simulink model "SF003A_Dampg"  (R2013b)
settings: Solver=FixedStepDiscrete  SolverMode=SingleTasking  StartTime=0.0  StopTime=1  FixedStep=.002  RelTol=1e-3
values from neighbouring files (symbols this model uses):
  ARCHGLBPRM_2MILLISEC_SEC_F32 = DataDict.Constant    [SF003A_Dampg_DataDict.m]
  DampgHydBasCoeff1 = DataDict.Calibration    [SF003A_Dampg_DataDict.m]
  DampgHydBasCoeff2 = DataDict.Calibration    [SF003A_Dampg_DataDict.m]
  DampgHydBasCoeff3 = DataDict.Calibration    [SF003A_Dampg_DataDict.m]
  DampgHydBasCoeff4 = DataDict.Calibration    [SF003A_Dampg_DataDict.m]
  DampgHydOutpLim = DataDict.Calibration    [SF003A_Dampg_DataDict.m]
  DampgQuad13Mplr = DataDict.Calibration    [SF003A_Dampg_DataDict.m]
  DampgQuad24Mplr = DataDict.Calibration    [SF003A_Dampg_DataDict.m]
  DampgQuadHwTqBacklsh = DataDict.Calibration    [SF003A_Dampg_DataDict.m]
  DampgQuadMotVelBacklsh = DataDict.Calibration    [SF003A_Dampg_DataDict.m]
  FLTINJ_DAMPG_DAMPGCMDBAS = DataDict.Constant    [SF003A_Dampg_DataDict.m]
libraries: FloatToFixd x9, Fil x8, FixdToFloat x8, LnrIntrpn x7, NxtrAbslt x5, NxtrSign x3, NxtrLim x3, simulink x1, NxtrMax x1, BilnrIntrpnMplX x1
(part 1 of 2)
settings Model: Creator=TZ5743  LastModifiedBy=bzhf94
settings SolverCC: AutoInsertRateTranBlk=on  InsertRTBMode=Always
settings DataIOCC: LimitDataPoints=off  SaveFormat=Structure  ReturnWorkspaceOutputs=on
settings OptimizationCC: BlockReduction=off  InlineParams=on  ZeroExternalMemoryAtStartup=off  ZeroInternalMemoryAtStartup=off  OptimizeModelRefInitCode=on  LifeSpan=1
settings DebuggingCC: SignalInfNanChecking=error  SignalRangeChecking=warning  UnderspecifiedInitializationDetection=Simplified  SolverPrmCheckMsg=error  InheritedTsInSrcMsg=error  DiscreteInheritContinuousMsg=error  SingleTaskRateTransMsg=error  TasksWithSamePriorityMsg=error  SigSpecEnsureSampleTimeMsg=error  CheckMatrixSingularityMsg=error  ParameterUnderflowMsg=error  ParameterPrecisionLossMsg=error  ParameterTunabilityLossMsg=error  FixptConstUnderflowMsg=warning  FixptConstOverflowMsg=warning  VectorMatrixConversionMsg=error  SignalLabelMismatchMsg=error  UnconnectedInputMsg=error  UnconnectedOutputMsg=error  UnconnectedLineMsg=error  SFcnCompatibilityMsg=error  UniqueDataStoreMsg=warning  BusObjectLabelMismatch=error  RootOutportRequireBusObject=error  AssertControl=DisableAll  ModelReferenceIOMsg=error  ModelReferenceVersionMismatchMessage=warning  ModelReferenceIOMismatchMessage=error  ModelReferenceCSMismatchMessage=warning  ModelReferenceDataLoggingMessage=error  StateNameClashWarn=warning  StrictBusMsg=ErrorOnBusTreatedAsVector  NonBusSignalsTreatedAsBus=error  SFUnexpectedBacktrackingDiag=error  SFInvalidInputDataAccessInChartInitDiag=error  SFNoUnconditionalDefaultTransitionDiag=error  SFTransitionOutsideNaturalParentDiag=error  SFUnconditionalTransitionShadowingDiag=error  SFUndirectedBroadcastEventsDiag=error
settings ModelReferenceCC: ModelReferenceNumInstancesAllowed=Single
settings RTWCC: SystemTargetFile=autosar.tlc  GenCodeOnly=on  TemplateMakefile=ert_default_tmf  Description=AUTOSAR  GenerateReport=on  ProcessScript=autosar_make_rtw_hook  LaunchReport=on
settings CodeAppCC: GenerateComments=off  IgnoreCustomStorageClasses=off  CustomSymbolStrType=$N$R$M  CustomSymbolStrBlkIO=$N$M  SimulinkBlockComments=off
settings STFCustomTargetCC: ParMdlRefBuildCompliant=on  CompOptLevelCompliant=on  IncludeMdlTerminateFcn=off  CombineOutputUpdateFcns=on  SuppressErrorStatus=on  ERTFirstTimeCompliant=on  ERTCustomFileBanners=on  SupportNonFinite=off  SupportComplex=off  SupportContinuousTime=off  SupportNonInlinedSFcns=off  MATLABClassNameForMDSCustomization=Simulink.SoftwareTarget.ERTCustomization  AutosarCompliant=on  GRTInterface=off  SystemTargetFile=autosar.tlc
settings ERTTargetCC: CodeReplacementLibrary=ANSI_C  ConcurrentExecutionCompliant=off  IncludeMdlTerminateFcn=off  SuppressErrorStatus=on  SupportNonFinite=off  SupportComplex=off  ModelStepFunctionPrototypeControlCompliant=off  CPPClassGenCompliant=off  AutosarCompliant=on  InlinedParameterPlacement=NonHierarchical  ERTCustomFileTemplate=example_file_process.tlc  EnableUserReplacementTypes=on

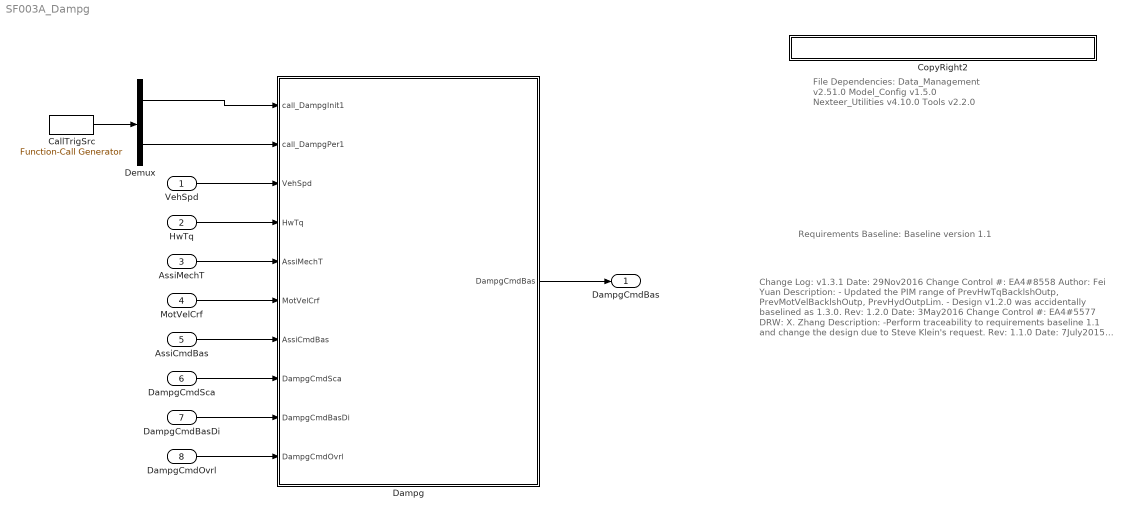
== system SF003A_Dampg ==
  note: File Dependencies:
      |
      | Data_Management v2.51.0
      | Model_Config v1.5.0
      | Nexteer_Utilities v4.10.0
      | Tools v2.2.0
  note: Requirements Baseline: Baseline version 1.1
  note: Change Log:
      |
      | v1.3.1
      | Date: 29Nov2016
      | Change Control #: EA4#8558
      | Author: Fei Yuan
      | Description:
      | - Updated the PIM range of PrevHwTqBacklshOutp,
      |   PrevMotVelBacklshOutp, PrevHydOutpLim.
      | - Design v1.2.0 was accidentally baselined as 1.3.0.
      |
      |
      | Rev: 1.2.0
      | Date: 3May2016
      | Change Control #: EA4#5577
      | DRW: X. Zhang
      | Description:
      | -Perform traceability to requirements baseline 1.1
      | and change the design due to Steve Klein's request.
      |
      | Rev: 1.1.0
      | Date: 7July2015
      | Change Control #: EA4#762
      | DRW: Sudeep Shankar
      | Description:
      | - Design update from EA3 to EA4 with data dictionary
      | changes.
      |
      |
      | v1.0.0
      | Date: 24-Jun-2015
      | Change Control #: EA4#762
      | DRW:  Sudeep Shankar
      | Description:
      | - Initial Release based off of EA3 Version 009
  VehSpd : Inport  RequirementInfo={'linktype_rmi_doors' '0000a525 (/E-STEER Core/SubSystem Specifications/Application Functions/SF003A Damping)' '#SF003A_33' 'true' 'REQ: SF003A_33' '' } %GIDa_568c51fe_83b0_458b_bd6e_4be12eab579e
  HwTq : Inport  RequirementInfo={'linktype_rmi_doors' '0000a525 (/E-STEER Core/SubSystem Specifications/Application Functions/SF003A Damping)' '#SF003A_34' 'true' 'REQ: SF003A_34' '' } %GIDa_93ae967a_0df1_4d53_9d75_79742e7754a9  Port=2
  AssiMechT : Inport  RequirementInfo={'linktype_rmi_doors' '0000a525 (/E-STEER Core/SubSystem Specifications/Application Functions/SF003A Damping)' '#SF003A_35' 'true' 'REQ: SF003A_35' '' } %GIDa_1636facc_5bec_431d_9ade_0f003592cb00  Port=3
  MotVelCrf : Inport  RequirementInfo={'linktype_rmi_doors' '0000a525 (/E-STEER Core/SubSystem Specifications/Application Functions/SF003A Damping)' '#SF003A_36' 'true' 'REQ: SF003A_36' '' } %GIDa_f33306b7_8b32_4dca_8a0a_81a3a24a2a49  Port=4
  AssiCmdBas : Inport  RequirementInfo={'linktype_rmi_doors' '0000a525 (/E-STEER Core/SubSystem Specifications/Application Functions/SF003A Damping)' '#SF003A_37' 'true' 'REQ: SF003A_37' '' } %GIDa_bfde9b7a_b609_47ac_97d9_497bdc083739  Port=5
  DampgCmdSca : Inport  RequirementInfo={'linktype_rmi_doors' '0000a525 (/E-STEER Core/SubSystem Specifications/Application Functions/SF003A Damping)' '#SF003A_38' 'true' 'REQ: SF003A_38' '' } %GIDa_3f9e7f26_4227_4164_8f57_da4171e42017  Port=6
  DampgCmdBasDi : Inport  RequirementInfo={'linktype_rmi_doors' '0000a525 (/E-STEER Core/SubSystem Specifications/Application Functions/SF003A Damping)' '#SF003A_9' 'true' 'REQ: SF003A_9' '' } %GIDa_728ec3ad_7cb0_4a0a_ae43_e264b5abcd56  Port=7
  DampgCmdOvrl : Inport  RequirementInfo={'linktype_rmi_doors' '0000a525 (/E-STEER Core/SubSystem Specifications/Application Functions/SF003A Damping)' '#SF003A_63' 'true' 'REQ: SF003A_63' '' } %GIDa_4827e2e0_a4cb_4f02_b938_6d875c7b4f9b  Port=8
  CallTrigSrc : simulink/Ports & Subsystems/Function-Call Generator  RequirementInfo={} %GIDa_ba0e12fc_4474_4f55_8217_81b6c7a3534f  sample_time=0.002  numberOfIterations=1
  CopyRight2 : Subsystem  Description=|  mask(Copyright Information){none=on}
      | Copyright info block.                                               
      |                                                                     
      | Place copyright information at the top of every subsystem in design.
      mask prompts: none "No parameters"
      mask help: Place copyright information at the top of every subsystem in design.
      mask Display:
      | NxtrConf = 'Nexteer Confidential';
      | 
      | sys = bdroot; %handle for the current model ("system")
      | first = get_param(sys,'Created');
      | if(isempty(first))
      |     first = datestr(now,'yyyy');
      | else
      |     first = first(end-3:end);  %year is last four digits
      | end
      | 
      | last = get_param(sys,'LastModifiedDate');
      | if isempty(last)
      |     last = datestr(now,'yyyy');
      | else
      |     last = last(end-3:end);
      | end
      | 
      | if strcmp(first,last)
      |     fprintf('%s -- Copyright %s Nexteer',NxtrConf,first)
      | else
      |     fprintf('%s -- %s%s- %s Nexteer',NxtrConf,char(169),first,last)
      | end
  Dampg : Subsystem
  Demux : Demux  Outputs=2
  DampgCmdBas : Outport  RequirementInfo={'linktype_rmi_doors' '0000a525 (/E-STEER Core/SubSystem Specifications/Application Functions/SF003A Damping)' '#SF003A_11' 'true' 'REQ: SF003A_11' '' } %GIDa_820641fa_7a17_4c33_aa73_2ea523178ec1
  wires:
  Demux/2 -> Dampg/2(call_DampgPer1)
  VehSpd/1 -> Dampg/3(VehSpd)
  HwTq/1 -> Dampg/4(HwTq)
  AssiMechT/1 -> Dampg/5(AssiMechT)
  MotVelCrf/1 -> Dampg/6(MotVelCrf)
  AssiCmdBas/1 -> Dampg/7(AssiCmdBas)
  DampgCmdSca/1 -> Dampg/8(DampgCmdSca)
  DampgCmdBasDi/1 -> Dampg/9(DampgCmdBasDi)
  DampgCmdOvrl/1 -> Dampg/10(DampgCmdOvrl)
  Dampg/1(DampgCmdBas) -> DampgCmdBas/1
  CallTrigSrc/1 -> Demux/1
  Demux/1 -> Dampg/1(call_DampgInit1)

== system SF003A_Dampg/CopyRight2 ==

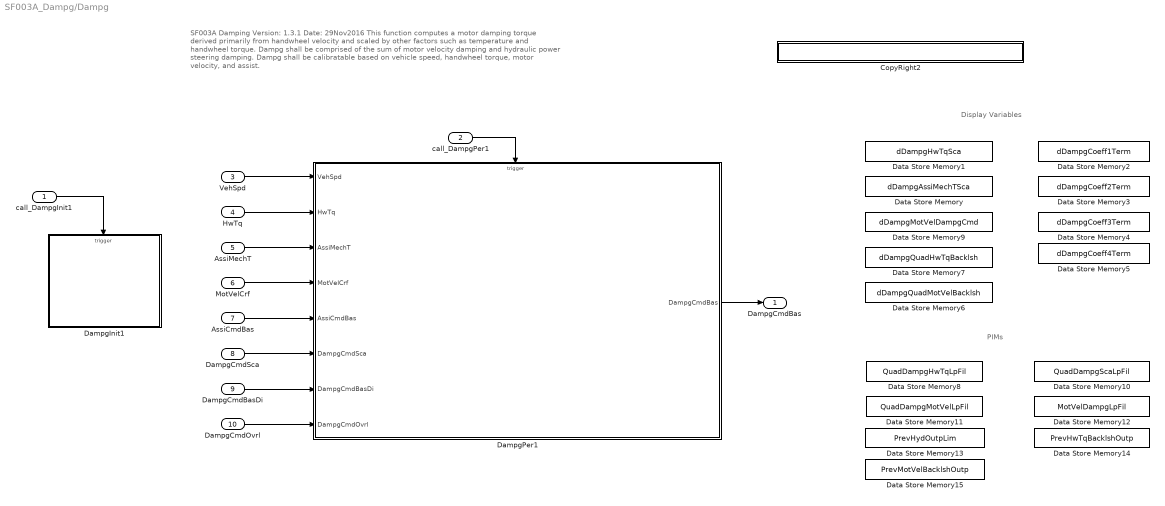
== system SF003A_Dampg/Dampg ==
  note: PIMs
  note: Display Variables
  note: SF003A Damping       Version: 1.3.1                                                      Date: 29Nov2016
      |
      | This function computes a motor damping torque derived primarily from handwheel velocity and scaled by other factors such as temperature and handwheel torque.
      | Dampg shall be comprised of the sum of motor velocity damping and hydraulic power steering damping.
      | Dampg shall be calibratable based on vehicle speed, handwheel torque, motor velocity, and assist.
  call_DampgInit1 : Inport
  call_DampgPer1 : Inport  Port=2
  VehSpd : Inport  Port=3
  HwTq : Inport  Port=4
  AssiMechT : Inport  Port=5
  MotVelCrf : Inport  Port=6
  AssiCmdBas : Inport  Port=7
  DampgCmdSca : Inport  Port=8
  DampgCmdBasDi : Inport  Port=9
  DampgCmdOvrl : Inport  Port=10
  CopyRight2 : Subsystem  Description=|  mask(Copyright Information){none=on}
      | Copyright info block.                                               
      |                                                                     
      | Place copyright information at the top of every subsystem in design.
      mask prompts: none "No parameters"
      mask help: Place copyright information at the top of every subsystem in design.
      mask Display:
      | NxtrConf = 'Nexteer Confidential';
      | 
      | sys = bdroot; %handle for the current model ("system")
      | first = get_param(sys,'Created');
      | if(isempty(first))
      |     first = datestr(now,'yyyy');
      | else
      |     first = first(end-3:end);  %year is last four digits
      | end
      | 
      | last = get_param(sys,'LastModifiedDate');
      | if isempty(last)
      |     last = datestr(now,'yyyy');
      | else
      |     last = last(end-3:end);
      | end
      | 
      | if strcmp(first,last)
      |     fprintf('%s -- Copyright %s Nexteer',NxtrConf,first)
      | else
      |     fprintf('%s -- %s%s- %s Nexteer',NxtrConf,char(169),first,last)
      | end
  DampgInit1 : Subsystem
  DampgPer1 : Subsystem
  Data Store Memory : DataStoreMemory  DataStoreName=dDampgAssiMechTSca  ReadBeforeWriteMsg=warning  WriteAfterWriteMsg=warning  WriteAfterReadMsg=warning  StateMustResolveToSignalObject=on
  Data Store Memory1 : DataStoreMemory  DataStoreName=dDampgHwTqSca  ReadBeforeWriteMsg=warning  WriteAfterWriteMsg=warning  WriteAfterReadMsg=warning  OutDataTypeStr=single  StateMustResolveToSignalObject=on
  Data Store Memory10 : DataStoreMemory  DataStoreName=QuadDampgScaLpFil  InitialValue=struct('FilSt',single(0),'FilGain',single(0))  OutDataTypeStr=Bus: FilLpRec1  StateMustResolveToSignalObject=on
  Data Store Memory11 : DataStoreMemory  DataStoreName=QuadDampgMotVelLpFil  InitialValue=struct('FilSt',single(0),'FilGain',single(0))  OutDataTypeStr=Bus: FilLpRec1  StateMustResolveToSignalObject=on
  Data Store Memory12 : DataStoreMemory  DataStoreName=MotVelDampgLpFil  InitialValue=struct('FilSt',single(0),'FilGain',single(0))  OutDataTypeStr=Bus: FilLpRec1  StateMustResolveToSignalObject=on
  Data Store Memory13 : DataStoreMemory  DataStoreName=PrevHydOutpLim  StateMustResolveToSignalObject=on
  Data Store Memory14 : DataStoreMemory  DataStoreName=PrevHwTqBacklshOutp  StateMustResolveToSignalObject=on
  Data Store Memory15 : DataStoreMemory  DataStoreName=PrevMotVelBacklshOutp  StateMustResolveToSignalObject=on
  Data Store Memory2 : DataStoreMemory  DataStoreName=dDampgCoeff1Term  ReadBeforeWriteMsg=warning  WriteAfterWriteMsg=warning  WriteAfterReadMsg=warning  OutDataTypeStr=single  StateMustResolveToSignalObject=on
  Data Store Memory3 : DataStoreMemory  DataStoreName=dDampgCoeff2Term  ReadBeforeWriteMsg=warning  WriteAfterWriteMsg=warning  WriteAfterReadMsg=warning  OutDataTypeStr=single  StateMustResolveToSignalObject=on
  Data Store Memory4 : DataStoreMemory  DataStoreName=dDampgCoeff3Term  ReadBeforeWriteMsg=warning  WriteAfterWriteMsg=warning  WriteAfterReadMsg=warning  OutDataTypeStr=single  StateMustResolveToSignalObject=on
  Data Store Memory5 : DataStoreMemory  DataStoreName=dDampgCoeff4Term  ReadBeforeWriteMsg=warning  WriteAfterWriteMsg=warning  WriteAfterReadMsg=warning  OutDataTypeStr=single  StateMustResolveToSignalObject=on
  Data Store Memory6 : DataStoreMemory  DataStoreName=dDampgQuadMotVelBacklsh  ReadBeforeWriteMsg=warning  WriteAfterWriteMsg=warning  WriteAfterReadMsg=warning  StateMustResolveToSignalObject=on
  Data Store Memory7 : DataStoreMemory  DataStoreName=dDampgQuadHwTqBacklsh  ReadBeforeWriteMsg=warning  WriteAfterWriteMsg=warning  WriteAfterReadMsg=warning  StateMustResolveToSignalObject=on
  Data Store Memory8 : DataStoreMemory  DataStoreName=QuadDampgHwTqLpFil  InitialValue=struct('FilSt',single(0),'FilGain',single(0))  OutDataTypeStr=Bus: FilLpRec1  StateMustResolveToSignalObject=on
  Data Store Memory9 : DataStoreMemory  DataStoreName=dDampgMotVelDampgCmd  ReadBeforeWriteMsg=warning  WriteAfterWriteMsg=warning  WriteAfterReadMsg=warning  StateMustResolveToSignalObject=on
  DampgCmdBas : Outport
  wires:
  MotVelCrf/1 -> DampgPer1/4(MotVelCrf)
  DampgCmdBasDi/1 -> DampgPer1/7(DampgCmdBasDi)
  DampgPer1/1(DampgCmdBas) -> DampgCmdBas/1
  DampgCmdSca/1 -> DampgPer1/6(DampgCmdSca)
  AssiMechT/1 -> DampgPer1/3(AssiMechT)
  DampgCmdOvrl/1 -> DampgPer1/8(DampgCmdOvrl)
  HwTq/1 -> DampgPer1/2(HwTq)
  AssiCmdBas/1 -> DampgPer1/5(AssiCmdBas)
  VehSpd/1 -> DampgPer1/1(VehSpd)
  call_DampgPer1/1 -> DampgPer1/Trigger
  call_DampgInit1/1 -> DampgInit1/Trigger

== system SF003A_Dampg/Dampg/CopyRight2 ==

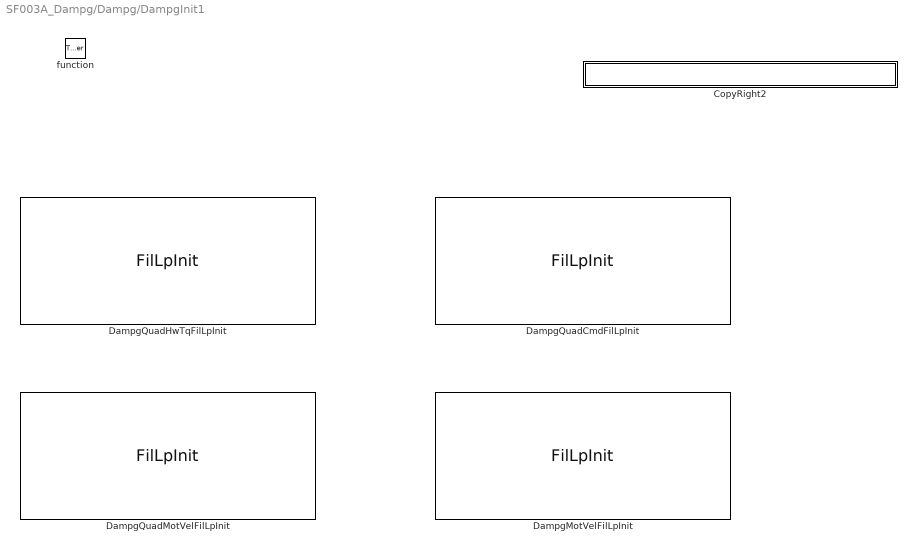
== system SF003A_Dampg/Dampg/DampgInit1 ==
  function : TriggerPort  TriggerType=function-call
  CopyRight2 : Subsystem  Description=|  mask(Copyright Information){none=on}
      | Copyright info block.                                               
      |                                                                     
      | Place copyright information at the top of every subsystem in design.
      mask prompts: none "No parameters"
      mask help: Place copyright information at the top of every subsystem in design.
      mask Display:
      | NxtrConf = 'Nexteer Confidential';
      | 
      | sys = bdroot; %handle for the current model ("system")
      | first = get_param(sys,'Created');
      | if(isempty(first))
      |     first = datestr(now,'yyyy');
      | else
      |     first = first(end-3:end);  %year is last four digits
      | end
      | 
      | last = get_param(sys,'LastModifiedDate');
      | if isempty(last)
      |     last = datestr(now,'yyyy');
      | else
      |     last = last(end-3:end);
      | end
      | 
      | if strcmp(first,last)
      |     fprintf('%s -- Copyright %s Nexteer',NxtrConf,first)
      | else
      |     fprintf('%s -- %s%s- %s Nexteer',NxtrConf,char(169),first,last)
      | end
  DampgMotVelFilLpInit : Fil/FilLpInit  Ic=0  Ts=ARCHGLBPRM_2MILLISEC_SEC_F32  Freq=DampgMotVelLpFilFrq  StVar=MotVelDampgLpFil
  DampgQuadCmdFilLpInit : Fil/FilLpInit  Ic=0  Ts=ARCHGLBPRM_2MILLISEC_SEC_F32  Freq=DampgQuadScaLpFilFrq  StVar=QuadDampgScaLpFil
  DampgQuadHwTqFilLpInit : Fil/FilLpInit  Ic=0  Ts=ARCHGLBPRM_2MILLISEC_SEC_F32  Freq=DampgQuadHwTqLpFilFrq  StVar=QuadDampgHwTqLpFil
  DampgQuadMotVelFilLpInit : Fil/FilLpInit  Ic=0  Ts=ARCHGLBPRM_2MILLISEC_SEC_F32  Freq=DampgQuadMotVelLpFilFrq  StVar=QuadDampgMotVelLpFil

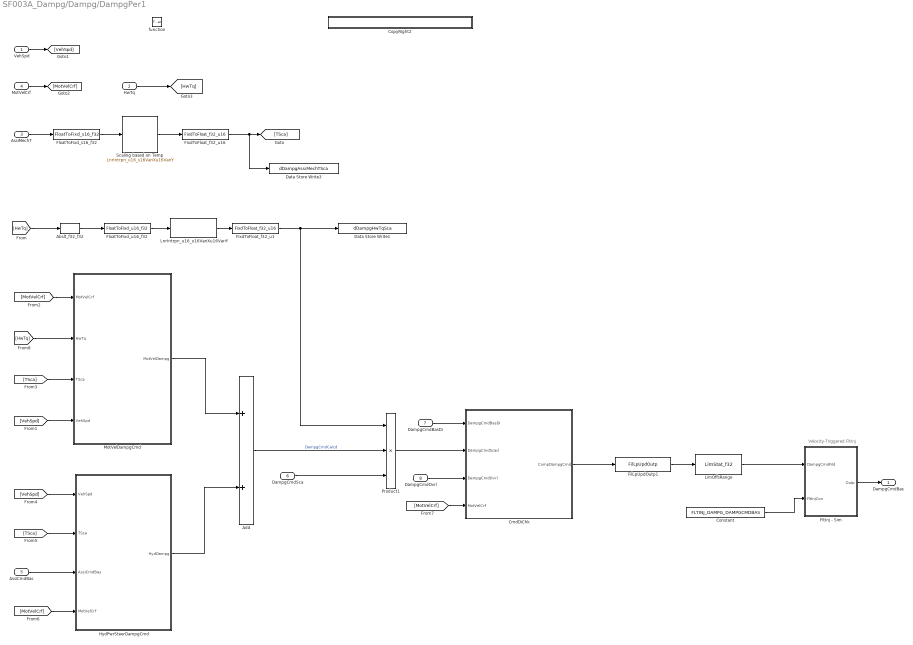
== system SF003A_Dampg/Dampg/DampgPer1 ==
  note: Velocity-Triggered FltInj
  VehSpd : Inport
  HwTq : Inport  Port=2
  AssiMechT : Inport  RequirementInfo={'linktype_rmi_doors' '0000a525 (/E-STEER Core/SubSystem Specifications/Application Functions/SF003A Damping)' '#SF003A_83' 'true' 'REQ: SF003A_83' '' } %GIDa_7550e755_adaf_43cd_af46_c12af1f44501  Port=3
  MotVelCrf : Inport  Port=4
  AssiCmdBas : Inport  Port=5
  DampgCmdSca : Inport  Port=6
  DampgCmdBasDi : Inport  Port=7
  DampgCmdOvrl : Inport  Port=8
  function : TriggerPort  TriggerType=function-call
  Abslt_f32_f32 : NxtrAbslt/Abslt_f32_f32  RequirementInfo={'linktype_rmi_doors' '0000a525 (/E-STEER Core/SubSystem Specifications/Application Functions/SF003A Damping)' '#SF003A_93' 'true' 'REQ: SF003A_93' '' } %GIDa_152aa55c_ff3e_4795_aeae_1a4fd5587628  SFunctionSpec=single y1 = Abslt_f32_f32(single u1)
      settings: AttributesFormatString=%<Name>
  Add : Sum  RequirementInfo={'linktype_rmi_doors' '0000a525 (/E-STEER Core/SubSystem Specifications/Application Functions/SF003A Damping)' '#SF003A_125' 'true' 'REQ: SF003A_125' '' } %GIDa_a51e37c2_da29_4b95_a7c8_8c19c8d9e4f2
  CmdDiChk : Subsystem
  Constant : Constant  Value=FLTINJ_DAMPG_DAMPGCMDBAS
  CopyRight2 : Subsystem  Description=|  mask(Copyright Information){none=on}
      | Copyright info block.                                               
      |                                                                     
      | Place copyright information at the top of every subsystem in design.
      mask prompts: none "No parameters"
      mask help: Place copyright information at the top of every subsystem in design.
      mask Display:
      | NxtrConf = 'Nexteer Confidential';
      | 
      | sys = bdroot; %handle for the current model ("system")
      | first = get_param(sys,'Created');
      | if(isempty(first))
      |     first = datestr(now,'yyyy');
      | else
      |     first = first(end-3:end);  %year is last four digits
      | end
      | 
      | last = get_param(sys,'LastModifiedDate');
      | if isempty(last)
      |     last = datestr(now,'yyyy');
      | else
      |     last = last(end-3:end);
      | end
      | 
      | if strcmp(first,last)
      |     fprintf('%s -- Copyright %s Nexteer',NxtrConf,first)
      | else
      |     fprintf('%s -- %s%s- %s Nexteer',NxtrConf,char(169),first,last)
      | end
  Data Store Write1 : DataStoreWrite  DataStoreName=dDampgHwTqSca
  Data Store Write3 : DataStoreWrite  DataStoreName=dDampgAssiMechTSca
  FilLpUpdOutp1 : Fil/FilLpUpdOutp  RequirementInfo={'linktype_rmi_doors' '0000a525 (/E-STEER Core/SubSystem Specifications/Application Functions/SF003A Damping)' '#SF003A_130' 'true' 'REQ: SF003A_130' '' } %GIDa_9b76992c_6716_46d2_8232_6364667a20c4  StVar=MotVelDampgLpFil
      settings: AttributesFormatString=StVar: %<StVar>
  FixdToFloat_f32_u1 : FixdToFloat/FixdToFloat_f32_u16  RequirementInfo={'linktype_rmi_doors' '0000a525 (/E-STEER Core/SubSystem Specifications/Application Functions/SF003A Damping)' '#SF003A_93' 'true' 'REQ: SF003A_93' '' } %GIDa_93b5cec2_bcdc_4944_b939_7a0cd5e9fed0  Param1=15
  FixdToFloat_f32_u16 : FixdToFloat/FixdToFloat_f32_u16  RequirementInfo={'linktype_rmi_doors' '0000a525 (/E-STEER Core/SubSystem Specifications/Application Functions/SF003A Damping)' '#SF003A_83' 'true' 'REQ: SF003A_83' '' } %GIDa_983a16aa_5c94_4ecb_93d6_d25a8d58e50a  Param1=12
  FloatToFixd_s16_f32 : FloatToFixd/FloatToFixd_s16_f32  RequirementInfo={'linktype_rmi_doors' '0000a525 (/E-STEER Core/SubSystem Specifications/Application Functions/SF003A Damping)' '#SF003A_83' 'true' 'REQ: SF003A_83' '' } %GIDa_f83f1ff1_03e3_4238_8bb3_25bc87451b9b  Param1=7
  FloatToFixd_u16_f32 : FloatToFixd/FloatToFixd_u16_f32  RequirementInfo={'linktype_rmi_doors' '0000a525 (/E-STEER Core/SubSystem Specifications/Application Functions/SF003A Damping)' '#SF003A_93' 'true' 'REQ: SF003A_93' '' } %GIDa_9d01660a_d186_40b6_83ad_ef8a565f4b3d  Param1=8
  FltInj - Sim : Subsystem  TreatAsAtomicUnit=on  VariantControl=FltInj_sim  mask(Fault_Injection){}
      mask help: Fault Injection is a simulation only block for EA4 programs.
  HydPwrSteerDampgCmd : Subsystem
  LimOffsRange : NxtrLim/LimStat_f32  RequirementInfo={'linktype_rmi_doors' '0000a525 (/E-STEER Core/SubSystem Specifications/Application Functions/SF003A Damping)' '#SF003A_131' 'true' 'REQ: SF003A_131' '' } %GIDa_822a07d5_0f05_4298_8afc_97f880dca36e  LoLim=SYSGLBPRM_MOTTQCMDLOLIM_MOTNWTMTR_F32  HiLim=SYSGLBPRM_MOTTQCMDHILIM_MOTNWTMTR_F32
      settings: AttributesFormatString=|
      | Low Limit: %<LoLim>
      | High Limit:%<HiLim>
  LnrIntrpn_u16_u16VariXu16VariY : LnrIntrpn/LnrIntrpn_u16_u16VariXu16VariY  RequirementInfo={'linktype_rmi_doors' '0000a525 (/E-STEER Core/SubSystem Specifications/Application Functions/SF003A Damping)' '#SF003A_93' 'true' 'REQ: SF003A_93' '' } %GIDa_b3e63933_aa2e_4fdf_a46c_c146a010da00  XTbl=DampgHwTqX  YTbl=DampgHwTqY
      settings: AttributesFormatString=Lnr ( u16VariX , u16VariY )
  MotVelDampgCmd : Subsystem
  Product1 : Product  RequirementInfo={'linktype_rmi_doors' '0000a525 (/E-STEER Core/SubSystem Specifications/Application Functions/SF003A Damping)' '#SF003A_126' 'true' 'REQ: SF003A_126' '' } %GIDa_ea32ba7a_0ccc_4c1b_8193_7b5dfbd1e212  Inputs=3  RndMeth=Zero
  Scaling based on Temp : LnrIntrpn/LnrIntrpn_u16_s16VariXu16VariY  RequirementInfo={'linktype_rmi_doors' '0000a525 (/E-STEER Core/SubSystem Specifications/Application Functions/SF003A Damping)' '#SF003A_83' 'true' 'REQ: SF003A_83' '' } %GIDa_d6c5a0d2_c9b9_4dbb_9c7f_b096228439d7  XTbl=DampgTScaX  YTbl=DampgTScaY
      settings: AttributesFormatString=Lnr ( s16VariX , u16VariY )
  DampgCmdBas : Outport
  wires:
  Constant/1 -> FltInj - Sim/2(FltInjCon)
  FltInj - Sim/1(Outp) -> DampgCmdBas/1
  Product1/1 -> CmdDiChk/2(DampgCmdScad)
  CmdDiChk/1(CompDampgCmd) -> FilLpUpdOutp1/1
  DampgCmdOvrl/1 -> CmdDiChk/3(DampgCmdOvrl)
  DampgCmdBasDi/1 -> CmdDiChk/1(DampgCmdBasDi)
  LimOffsRange/1 -> FltInj - Sim/1(DampgCmdFild)
  Scaling based on Temp/1 -> FixdToFloat_f32_u16/1
  AssiMechT/1 -> FloatToFixd_s16_f32/1
  FloatToFixd_s16_f32/1 -> Scaling based on Temp/1
  FixdToFloat_f32_u16/1 -> Data Store Write3/1, [TSca]
  VehSpd/1 -> [VehSpd]
  MotVelCrf/1 -> [MotVelCrf]
  [MotVelCrf] -> MotVelDampgCmd/1(MotVelCrf)
  [VehSpd] -> MotVelDampgCmd/4(VehSpd)
  [TSca] -> MotVelDampgCmd/3(TSca)
  [VehSpd] -> HydPwrSteerDampgCmd/1(VehSpd)
  [TSca] -> HydPwrSteerDampgCmd/2(TSca)
  AssiCmdBas/1 -> HydPwrSteerDampgCmd/3(AssiCmdBas)
  [MotVelCrf] -> HydPwrSteerDampgCmd/4(MotVelCrf)
  HydPwrSteerDampgCmd/1(HydDampg) -> Add/2
  MotVelDampgCmd/1(MotVelDampg) -> Add/1
  Add/1 -> Product1/2  "DampgCmdCalcd"
  DampgCmdSca/1 -> Product1/3
  [MotVelCrf] -> CmdDiChk/4(MotVelCrf)
  FilLpUpdOutp1/1 -> LimOffsRange/1
  FloatToFixd_u16_f32/1 -> LnrIntrpn_u16_u16VariXu16VariY/1
  LnrIntrpn_u16_u16VariXu16VariY/1 -> FixdToFloat_f32_u1/1
  FixdToFloat_f32_u1/1 -> Product1/1, Data Store Write1/1
  Abslt_f32_f32/1 -> FloatToFixd_u16_f32/1
  HwTq/1 -> [HwTq]
  [HwTq] -> Abslt_f32_f32/1
  [HwTq] -> MotVelDampgCmd/2(HwTq)

== system SF003A_Dampg/Dampg/DampgInit1/CopyRight2 ==

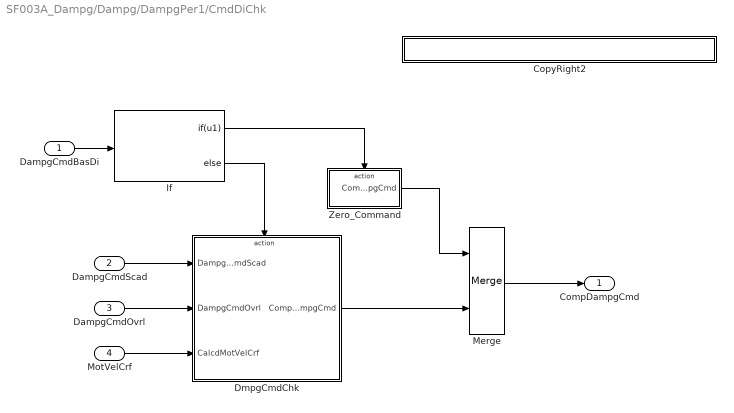
== system SF003A_Dampg/Dampg/DampgPer1/CmdDiChk ==
  DampgCmdBasDi : Inport
  DampgCmdScad : Inport  Port=2
  DampgCmdOvrl : Inport  Port=3
  MotVelCrf : Inport  Port=4
  CopyRight2 : Subsystem  Description=|  mask(Copyright Information){none=on}
      | Copyright info block.                                               
      |                                                                     
      | Place copyright information at the top of every subsystem in design.
      mask prompts: none "No parameters"
      mask help: Place copyright information at the top of every subsystem in design.
      mask Display:
      | NxtrConf = 'Nexteer Confidential';
      | 
      | sys = bdroot; %handle for the current model ("system")
      | first = get_param(sys,'Created');
      | if(isempty(first))
      |     first = datestr(now,'yyyy');
      | else
      |     first = first(end-3:end);  %year is last four digits
      | end
      | 
      | last = get_param(sys,'LastModifiedDate');
      | if isempty(last)
      |     last = datestr(now,'yyyy');
      | else
      |     last = last(end-3:end);
      | end
      | 
      | if strcmp(first,last)
      |     fprintf('%s -- Copyright %s Nexteer',NxtrConf,first)
      | else
      |     fprintf('%s -- %s%s- %s Nexteer',NxtrConf,char(169),first,last)
      | end
  DmpgCmdChk : Subsystem  RequirementInfo={} %GIDa_42609f80_721e_4222_a854_978db5b32e82  TreatAsAtomicUnit=on
  If : If  RequirementInfo={} %GIDa_e8daf89a_735d_4ce3_8883_6d943d5da402  IfExpression=u1
  Merge : Merge
  Zero_Command : Subsystem  RequirementInfo={'linktype_rmi_doors' '0000a525 (/E-STEER Core/SubSystem Specifications/Application Functions/SF003A Damping)' '#SF003A_127' 'true' 'REQ: SF003A_127' '' } %GIDa_8150363f_e871_4e58_837a_c9fd5c39bb6f  TreatAsAtomicUnit=on
  CompDampgCmd : Outport
  wires:
  If/2 -> DmpgCmdChk/Action
  If/1 -> Zero_Command/Action
  DampgCmdScad/1 -> DmpgCmdChk/1(DampgCmdScad)
  DmpgCmdChk/1(CompDampgCmd) -> Merge/2
  Zero_Command/1(CompDampgCmd) -> Merge/1
  Merge/1 -> CompDampgCmd/1
  DampgCmdBasDi/1 -> If/1
  DampgCmdOvrl/1 -> DmpgCmdChk/2(DampgCmdOvrl)
  MotVelCrf/1 -> DmpgCmdChk/3(CalcdMotVelCrf)

== system SF003A_Dampg/Dampg/DampgPer1/CopyRight2 ==

== system SF003A_Dampg/Dampg/DampgPer1/FltInj - Sim ==
  note: Inport #2 must be Constant
  note: EA4.x Fault Injection
  note: This block requires no modification by FDD author.
      |
      | This block does not actually simulate any fault injection.  It is simply a pass-thru.
      |
      | The port (#2) simply terminates its signal, but we are trying to force the FDD author
      | to properly use the Constant in FDD model.
  DampgCmdFild : Inport
  FltInjCon : Inport  Port=2
  CopyRight2 : Subsystem  Description=|  mask(Copyright Information){none=on}
      | Copyright info block.                                               
      |                                                                     
      | Place copyright information at the top of every subsystem in design.
      mask prompts: none "No parameters"
      mask help: Place copyright information at the top of every subsystem in design.
      mask Display:
      | NxtrConf = 'Nexteer Confidential';
      | 
      | sys = bdroot; %handle for the current model ("system")
      | first = get_param(sys,'Created');
      | if(isempty(first))
      |     first = datestr(now,'yyyy');
      | else
      |     first = first(end-3:end);  %year is last four digits
      | end
      | 
      | last = get_param(sys,'LastModifiedDate');
      | if isempty(last)
      |     last = datestr(now,'yyyy');
      | else
      |     last = last(end-3:end);
      | end
      | 
      | if strcmp(first,last)
      |     fprintf('%s -- Copyright %s Nexteer',NxtrConf,first)
      | else
      |     fprintf('%s -- %s%s- %s Nexteer',NxtrConf,char(169),first,last)
      | end
  Terminator : Terminator
  Outp : Outport
  wires:
  FltInjCon/1 -> Terminator/1
  DampgCmdFild/1 -> Outp/1

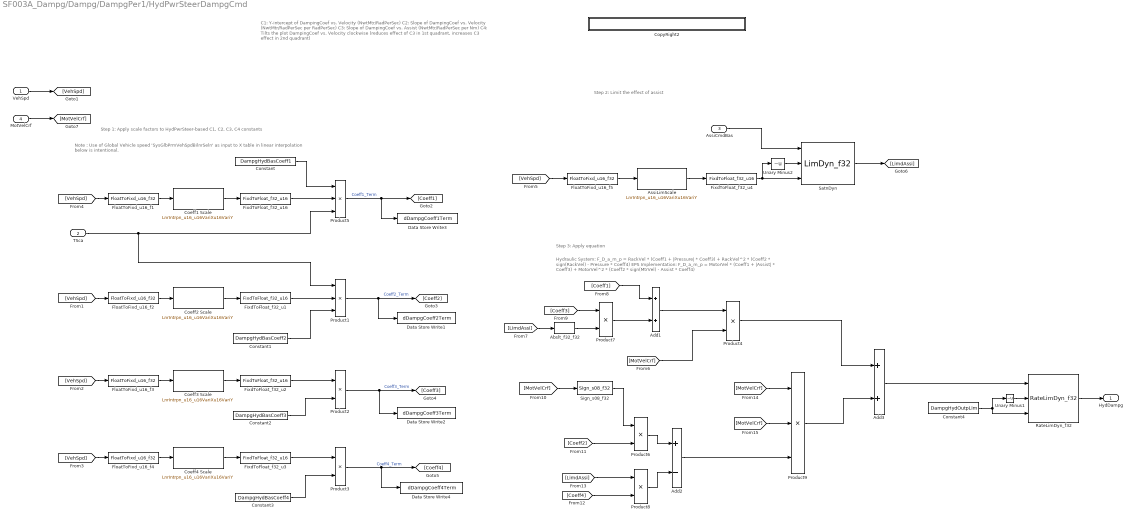
== system SF003A_Dampg/Dampg/DampgPer1/HydPwrSteerDampgCmd ==
  note: Note : Use of Global Vehicle speed 'SysGlbPrmVehSpdBilnrSeln' as input to X table in linear interpolation below is intentional.
  note: Hydraulic System:  F_D_a_m_p = RackVel * (Coeff1 + |Pressure| * Coeff3) + RackVel^2 * (Coeff2 * sign(RackVel) - Pressure * Coeff4)
      | EPS Implementation:  F_D_a_m_p = MotorVel * (Coeff1 + |Assist| * Coeff3) + MotorVel^2 * (Coeff2 * sign(MtrVel) - Assist * Coeff4)
  note: Step 3: Apply equation
  note: Step 2: Limit the effect of assist
  note: C1:  Y-intercept of DampingCoef vs. Velocity  (NwtMtr/RadPerSec)
      | C2:  Slope         of DampingCoef vs. Velocity  (NwtMtr/RadPerSec per RadPerSec)
      |
      | C3:  Slope         of DampingCoef vs. Assist      (NwtMtr/RadPerSec per Nm)
      | C4:  Tilts the plot   DampingCoef vs. Velocity clockwise (reduces effect of C3 in 1st quadrant, increases C3 effect in 2nd quadrant)
  note: Step 1: Apply scale factors to HydPwrSteer-based C1, C2, C3, C4 constants
  VehSpd : Inport
  TSca : Inport  Port=2
  AssiCmdBas : Inport  RequirementInfo={'linktype_rmi_doors' '0000a525 (/E-STEER Core/SubSystem Specifications/Application Functions/SF003A Damping)' '#SF003A_123' 'true' 'REQ: SF003A_123' '' } %GIDa_86305d61_c85b_4d27_94ee_c42e672ff448  Port=3
  MotVelCrf : Inport  Port=4
  Abslt_f32_f32 : NxtrAbslt/Abslt_f32_f32  RequirementInfo={'linktype_rmi_doors' '0000a525 (/E-STEER Core/SubSystem Specifications/Application Functions/SF003A Damping)' '#SF003A_134' 'true' 'REQ: SF003A_134' '' } %GIDa_f501944f_b822_4808_bbc9_5278a2863dba  SFunctionSpec=single y1 = Abslt_f32_f32(single u1)
      settings: AttributesFormatString=%<Name>
  Add1 : Sum  RequirementInfo={'linktype_rmi_doors' '0000a525 (/E-STEER Core/SubSystem Specifications/Application Functions/SF003A Damping)' '#SF003A_134' 'true' 'REQ: SF003A_134' '' } %GIDa_715c77c8_889f_48fb_bcdb_8e175ca2020c
  Add2 : Sum  RequirementInfo={'linktype_rmi_doors' '0000a525 (/E-STEER Core/SubSystem Specifications/Application Functions/SF003A Damping)' '#SF003A_134' 'true' 'REQ: SF003A_134' '' } %GIDa_08df5b53_9e8a_4b86_814f_98a1f87b8b16  Inputs=+-
  Add3 : Sum  RequirementInfo={'linktype_rmi_doors' '0000a525 (/E-STEER Core/SubSystem Specifications/Application Functions/SF003A Damping)' '#SF003A_134' 'true' 'REQ: SF003A_134' '' } %GIDa_4d1fb097_f55e_4c57_bdb9_4c1e69b47d24
  AssiLimScale : LnrIntrpn/LnrIntrpn_u16_u16VariXu16VariY  RequirementInfo={'linktype_rmi_doors' '0000a525 (/E-STEER Core/SubSystem Specifications/Application Functions/SF003A Damping)' '#SF003A_123' 'true' 'REQ: SF003A_123' '' } %GIDa_6bfd85c2_6315_461c_b996_b24c34637772  XTbl=SysGlbPrmVehSpdBilnrSeln  YTbl=DampgHydAssiLim
      settings: AttributesFormatString=Lnr ( u16VariX , u16VariY )
  Coeff1 Scale : LnrIntrpn/LnrIntrpn_u16_u16VariXu16VariY  RequirementInfo={'linktype_rmi_doors' '0000a525 (/E-STEER Core/SubSystem Specifications/Application Functions/SF003A Damping)' '#SF003A_119' 'true' 'REQ: SF003A_119' '' } %GIDa_e38cba12_2641_40e6_9d18_a448e9e7166a  XTbl=SysGlbPrmVehSpdBilnrSeln  YTbl=DampgHydCoeff1ScaY
      settings: AttributesFormatString=Lnr ( u16VariX , u16VariY )
  Coeff2 Scale : LnrIntrpn/LnrIntrpn_u16_u16VariXu16VariY  RequirementInfo={'linktype_rmi_doors' '0000a525 (/E-STEER Core/SubSystem Specifications/Application Functions/SF003A Damping)' '#SF003A_120' 'true' 'REQ: SF003A_120' '' } %GIDa_d24eb119_9d54_4127_8f49_7b8848458065  XTbl=SysGlbPrmVehSpdBilnrSeln  YTbl=DampgHydCoeff2ScaY
      settings: AttributesFormatString=Lnr ( u16VariX , u16VariY )
  Coeff3 Scale : LnrIntrpn/LnrIntrpn_u16_u16VariXu16VariY  RequirementInfo={'linktype_rmi_doors' '0000a525 (/E-STEER Core/SubSystem Specifications/Application Functions/SF003A Damping)' '#SF003A_121' 'true' 'REQ: SF003A_121' '' } %GIDa_72b39f25_b88e_49ed_8e35_1f932d582626  XTbl=SysGlbPrmVehSpdBilnrSeln  YTbl=DampgHydCoeff3ScaY
      settings: AttributesFormatString=Lnr ( u16VariX , u16VariY )
  Coeff4 Scale : LnrIntrpn/LnrIntrpn_u16_u16VariXu16VariY  RequirementInfo={'linktype_rmi_doors' '0000a525 (/E-STEER Core/SubSystem Specifications/Application Functions/SF003A Damping)' '#SF003A_122' 'true' 'REQ: SF003A_122' '' } %GIDa_d40d207a_a0cf_45d7_aac6_518a6c915d18  XTbl=SysGlbPrmVehSpdBilnrSeln  YTbl=DampgHydCoeff4ScaY
      settings: AttributesFormatString=Lnr ( u16VariX , u16VariY )
  Constant : Constant  RequirementInfo={'linktype_rmi_doors' '0000a525 (/E-STEER Core/SubSystem Specifications/Application Functions/SF003A Damping)' '#SF003A_119' 'true' 'REQ: SF003A_119' '' } %GIDa_e870ba0a_010e_468c_bd3d_22754f9fd79b  Value=DampgHydBasCoeff1
  Constant1 : Constant  RequirementInfo={'linktype_rmi_doors' '0000a525 (/E-STEER Core/SubSystem Specifications/Application Functions/SF003A Damping)' '#SF003A_120' 'true' 'REQ: SF003A_120' '' } %GIDa_0a0e34f7_b408_4cd2_bafe_d06fe50a73dd  Value=DampgHydBasCoeff2
  Constant2 : Constant  Value=DampgHydBasCoeff3
  Constant3 : Constant  Value=DampgHydBasCoeff4
  Constant4 : Constant  Value=DampgHydOutpLim
  CopyRight2 : Subsystem  Description=|  mask(Copyright Information){none=on}
      | Copyright info block.                                               
      |                                                                     
      | Place copyright information at the top of every subsystem in design.
      mask prompts: none "No parameters"
      mask help: Place copyright information at the top of every subsystem in design.
      mask Display:
      | NxtrConf = 'Nexteer Confidential';
      | 
      | sys = bdroot; %handle for the current model ("system")
      | first = get_param(sys,'Created');
      | if(isempty(first))
      |     first = datestr(now,'yyyy');
      | else
      |     first = first(end-3:end);  %year is last four digits
      | end
      | 
      | last = get_param(sys,'LastModifiedDate');
      | if isempty(last)
      |     last = datestr(now,'yyyy');
      | else
      |     last = last(end-3:end);
      | end
      | 
      | if strcmp(first,last)
      |     fprintf('%s -- Copyright %s Nexteer',NxtrConf,first)
      | else
      |     fprintf('%s -- %s%s- %s Nexteer',NxtrConf,char(169),first,last)
      | end
  Data Store Write1 : DataStoreWrite  DataStoreName=dDampgCoeff2Term
  Data Store Write2 : DataStoreWrite  DataStoreName=dDampgCoeff3Term
  Data Store Write3 : DataStoreWrite  DataStoreName=dDampgCoeff1Term
  Data Store Write4 : DataStoreWrite  DataStoreName=dDampgCoeff4Term
  FixdToFloat_f32_u1 : FixdToFloat/FixdToFloat_f32_u16  RequirementInfo={'linktype_rmi_doors' '0000a525 (/E-STEER Core/SubSystem Specifications/Application Functions/SF003A Damping)' '#SF003A_120' 'true' 'REQ: SF003A_120' '' } %GIDa_b47533fc_c7a2_479f_8c83_9c234aad9376  Param1=12
  FixdToFloat_f32_u16 : FixdToFloat/FixdToFloat_f32_u16  RequirementInfo={'linktype_rmi_doors' '0000a525 (/E-STEER Core/SubSystem Specifications/Application Functions/SF003A Damping)' '#SF003A_119' 'true' 'REQ: SF003A_119' '' } %GIDa_7dca0fd0_1b42_4f4c_bd4b_d82fe23ee9ba  Param1=12
  FixdToFloat_f32_u2 : FixdToFloat/FixdToFloat_f32_u16  RequirementInfo={'linktype_rmi_doors' '0000a525 (/E-STEER Core/SubSystem Specifications/Application Functions/SF003A Damping)' '#SF003A_121' 'true' 'REQ: SF003A_121' '' } %GIDa_57a67ce2_c6d8_469e_86ea_d293d5f31ace  Param1=12
  FixdToFloat_f32_u3 : FixdToFloat/FixdToFloat_f32_u16  RequirementInfo={'linktype_rmi_doors' '0000a525 (/E-STEER Core/SubSystem Specifications/Application Functions/SF003A Damping)' '#SF003A_122' 'true' 'REQ: SF003A_122' '' } %GIDa_aec6ab5d_f546_4e52_938e_919f10f346f2  Param1=12
  FixdToFloat_f32_u4 : FixdToFloat/FixdToFloat_f32_u16  RequirementInfo={'linktype_rmi_doors' '0000a525 (/E-STEER Core/SubSystem Specifications/Application Functions/SF003A Damping)' '#SF003A_123' 'true' 'REQ: SF003A_123' '' } %GIDa_fa603636_78d0_4317_a715_02eebae19e68  Param1=12
  FloatToFixd_u16_f1 : FloatToFixd/FloatToFixd_u16_f32  RequirementInfo={'linktype_rmi_doors' '0000a525 (/E-STEER Core/SubSystem Specifications/Application Functions/SF003A Damping)' '#SF003A_119' 'true' 'REQ: SF003A_119' '' } %GIDa_2c9b05d4_0aa1_4804_bb6f_b7aba2a66048  Param1=7
  FloatToFixd_u16_f2 : FloatToFixd/FloatToFixd_u16_f32  RequirementInfo={'linktype_rmi_doors' '0000a525 (/E-STEER Core/SubSystem Specifications/Application Functions/SF003A Damping)' '#SF003A_120' 'true' 'REQ: SF003A_120' '' } %GIDa_5e39595f_f68e_45d0_8b8d_3b49bfe7cb2c  Param1=7
  FloatToFixd_u16_f3 : FloatToFixd/FloatToFixd_u16_f32  RequirementInfo={'linktype_rmi_doors' '0000a525 (/E-STEER Core/SubSystem Specifications/Application Functions/SF003A Damping)' '#SF003A_121' 'true' 'REQ: SF003A_121' '' } %GIDa_d42f5a56_5f71_4771_8715_20fd48da2f1d  Param1=7
  FloatToFixd_u16_f4 : FloatToFixd/FloatToFixd_u16_f32  RequirementInfo={'linktype_rmi_doors' '0000a525 (/E-STEER Core/SubSystem Specifications/Application Functions/SF003A Damping)' '#SF003A_122' 'true' 'REQ: SF003A_122' '' } %GIDa_f91826a0_f8d6_4928_8826_05d0633d9a62  Param1=7
  FloatToFixd_u16_f5 : FloatToFixd/FloatToFixd_u16_f32  RequirementInfo={'linktype_rmi_doors' '0000a525 (/E-STEER Core/SubSystem Specifications/Application Functions/SF003A Damping)' '#SF003A_123' 'true' 'REQ: SF003A_123' '' } %GIDa_985b52ca_d61d_435c_a020_ea149c3807cc  Param1=7
  Product1 : Product  RequirementInfo={'linktype_rmi_doors' '0000a525 (/E-STEER Core/SubSystem Specifications/Application Functions/SF003A Damping)' '#SF003A_120' 'true' 'REQ: SF003A_120' '' } %GIDa_cb599213_e55b_4b7a_b605_d1e1f472c752  Inputs=3  RndMeth=Zero
  Product2 : Product  RequirementInfo={'linktype_rmi_doors' '0000a525 (/E-STEER Core/SubSystem Specifications/Application Functions/SF003A Damping)' '#SF003A_121' 'true' 'REQ: SF003A_121' '' } %GIDa_c7d07d79_c274_45f1_bd2f_c381ea8f0c68  RndMeth=Zero
  Product3 : Product  RequirementInfo={'linktype_rmi_doors' '0000a525 (/E-STEER Core/SubSystem Specifications/Application Functions/SF003A Damping)' '#SF003A_122' 'true' 'REQ: SF003A_122' '' } %GIDa_e4031464_97c0_4c31_ac40_0dd4d7c834ca  RndMeth=Zero
  Product4 : Product  RequirementInfo={'linktype_rmi_doors' '0000a525 (/E-STEER Core/SubSystem Specifications/Application Functions/SF003A Damping)' '#SF003A_134' 'true' 'REQ: SF003A_134' '' } %GIDa_42b4c2de_7cc3_40a0_b7b8_17eea4f9a20b  RndMeth=Zero
  Product5 : Product  RequirementInfo={'linktype_rmi_doors' '0000a525 (/E-STEER Core/SubSystem Specifications/Application Functions/SF003A Damping)' '#SF003A_119' 'true' 'REQ: SF003A_119' '' } %GIDa_7c73693c_e25d_402f_a7f2_104b7fea5ade  Inputs=3  RndMeth=Zero
  Product6 : Product  RequirementInfo={'linktype_rmi_doors' '0000a525 (/E-STEER Core/SubSystem Specifications/Application Functions/SF003A Damping)' '#SF003A_134' 'true' 'REQ: SF003A_134' '' } %GIDa_12b114f4_caef_47e2_9f75_351a92cdb420  RndMeth=Zero
  Product7 : Product  RequirementInfo={'linktype_rmi_doors' '0000a525 (/E-STEER Core/SubSystem Specifications/Application Functions/SF003A Damping)' '#SF003A_134' 'true' 'REQ: SF003A_134' '' } %GIDa_21290ff4_cdfa_4c0d_8524_1cdaa457b739  RndMeth=Zero
  Product8 : Product  RequirementInfo={'linktype_rmi_doors' '0000a525 (/E-STEER Core/SubSystem Specifications/Application Functions/SF003A Damping)' '#SF003A_134' 'true' 'REQ: SF003A_134' '' } %GIDa_b869f62b_5546_4f9d_a74f_346009d4c9bd  RndMeth=Zero
  Product9 : Product  RequirementInfo={'linktype_rmi_doors' '0000a525 (/E-STEER Core/SubSystem Specifications/Application Functions/SF003A Damping)' '#SF003A_134' 'true' 'REQ: SF003A_134' '' } %GIDa_bebd9314_41e9_4cbe_a469_d3ace663ff05  Inputs=3  RndMeth=Zero
  RateLimDyn_f32 : NxtrLim/RateLimDyn_f32  RequirementInfo={'linktype_rmi_doors' '0000a525 (/E-STEER Core/SubSystem Specifications/Application Functions/SF003A Damping)' '#SF003A_140' 'true' 'REQ: SF003A_140' '' } %GIDa_6384ec74_c73c_4bff_b5ee_e8a98ecf60bd  StVar=PrevHydOutpLim  Ts=ARCHGLBPRM_2MILLISEC_SEC_F32
      settings: AttributesFormatString=StVar: %<StVar>
  SatnDyn : NxtrLim/LimDyn_f32  RequirementInfo={'linktype_rmi_doors' '0000a525 (/E-STEER Core/SubSystem Specifications/Application Functions/SF003A Damping)' '#SF003A_123' 'true' 'REQ: SF003A_123' '' } %GIDa_21eff815_6580_4c93_9132_7c55a93ba868
  Sign_s08_f32 : NxtrSign/Sign_s08_f32  RequirementInfo={'linktype_rmi_doors' '0000a525 (/E-STEER Core/SubSystem Specifications/Application Functions/SF003A Damping)' '#SF003A_134' 'true' 'REQ: SF003A_134' '' } %GIDa_554b3242_045f_4c34_9734_1cf6d31e9673  SFunctionSpec=int8 y1 = Sign_s08_f32(single u1)
  Unary Minus1 : UnaryMinus
  Unary Minus2 : UnaryMinus  RequirementInfo={'linktype_rmi_doors' '0000a525 (/E-STEER Core/SubSystem Specifications/Application Functions/SF003A Damping)' '#SF003A_123' 'true' 'REQ: SF003A_123' '' } %GIDa_f223d2fe_e920_408c_ba84_cb10c6e4a170
  HydDampg : Outport
  wires:
  FloatToFixd_u16_f1/1 -> Coeff1 Scale/1
  Coeff1 Scale/1 -> FixdToFloat_f32_u16/1
  Constant/1 -> Product5/1
  TSca/1 -> Product5/3, Product1/1
  FixdToFloat_f32_u16/1 -> Product5/2
  Product5/1 -> Data Store Write3/1, [Coeff1]  "Coeff1_Term"
  VehSpd/1 -> [VehSpd]
  [VehSpd] -> FloatToFixd_u16_f1/1
  FloatToFixd_u16_f2/1 -> Coeff2 Scale/1
  Coeff2 Scale/1 -> FixdToFloat_f32_u1/1
  FixdToFloat_f32_u1/1 -> Product1/2
  Product1/1 -> Data Store Write1/1, [Coeff2]  "Coeff2_Term"
  [VehSpd] -> FloatToFixd_u16_f2/1
  Constant1/1 -> Product1/3
  FloatToFixd_u16_f3/1 -> Coeff3 Scale/1
  Coeff3 Scale/1 -> FixdToFloat_f32_u2/1
  FixdToFloat_f32_u2/1 -> Product2/1
  [VehSpd] -> FloatToFixd_u16_f3/1
  Constant2/1 -> Product2/2
  Product2/1 -> Data Store Write2/1, [Coeff3]  "Coeff3_Term"
  FloatToFixd_u16_f4/1 -> Coeff4 Scale/1
  Coeff4 Scale/1 -> FixdToFloat_f32_u3/1
  FixdToFloat_f32_u3/1 -> Product3/1
  [VehSpd] -> FloatToFixd_u16_f4/1
  Constant3/1 -> Product3/2
  Product3/1 -> Data Store Write4/1, [Coeff4]  "Coeff4_Term"
  [VehSpd] -> FloatToFixd_u16_f5/1
  FloatToFixd_u16_f5/1 -> AssiLimScale/1
  AssiCmdBas/1 -> SatnDyn/1
  AssiLimScale/1 -> FixdToFloat_f32_u4/1
  Unary Minus2/1 -> SatnDyn/2
  FixdToFloat_f32_u4/1 -> Unary Minus2/1, SatnDyn/3
  SatnDyn/1 -> [LimdAssi]
  MotVelCrf/1 -> [MotVelCrf]
  [MotVelCrf] -> Product4/2
  Product7/1 -> Add1/2
  [Coeff1] -> Add1/1
  [Coeff3] -> Product7/1
  [LimdAssi] -> Abslt_f32_f32/1
  Abslt_f32_f32/1 -> Product7/2
  Add1/1 -> Product4/1
  [MotVelCrf] -> Sign_s08_f32/1
  Sign_s08_f32/1 -> Product6/1
  [Coeff2] -> Product6/2
  [LimdAssi] -> Product8/1
  [Coeff4] -> Product8/2
  Product8/1 -> Add2/2
  Product6/1 -> Add2/1
  Add2/1 -> Product9/3
  [MotVelCrf] -> Product9/1
  [MotVelCrf] -> Product9/2
  Product4/1 -> Add3/1
  Product9/1 -> Add3/2
  Add3/1 -> RateLimDyn_f32/1
  RateLimDyn_f32/1 -> HydDampg/1
  Constant4/1 -> Unary Minus1/1, RateLimDyn_f32/3
  Unary Minus1/1 -> RateLimDyn_f32/2

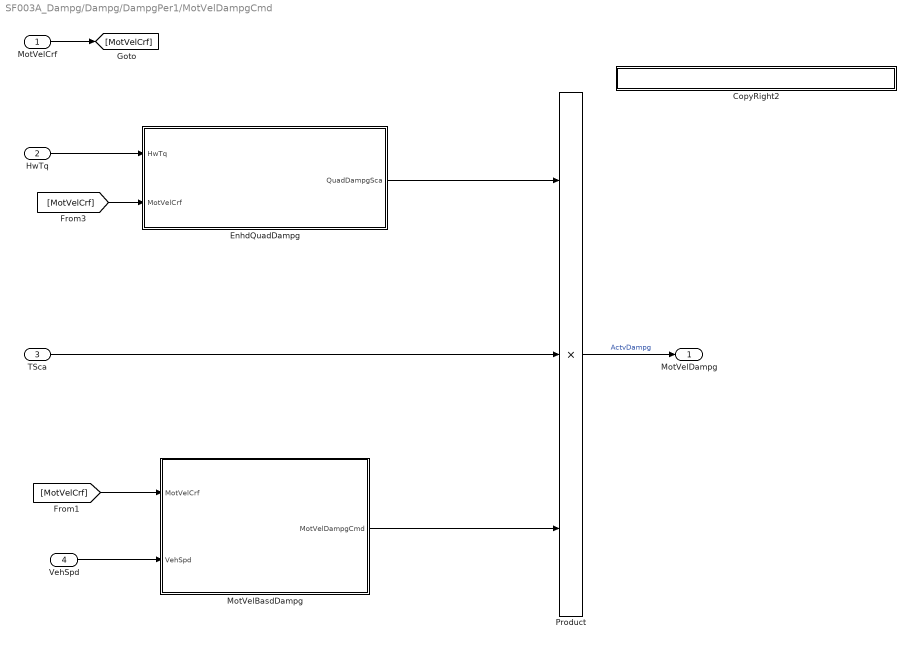
== system SF003A_Dampg/Dampg/DampgPer1/MotVelDampgCmd ==
  MotVelCrf : Inport
  HwTq : Inport  Port=2
  TSca : Inport  Port=3
  VehSpd : Inport  Port=4
  CopyRight2 : Subsystem  Description=|  mask(Copyright Information){none=on}
      | Copyright info block.                                               
      |                                                                     
      | Place copyright information at the top of every subsystem in design.
      mask prompts: none "No parameters"
      mask help: Place copyright information at the top of every subsystem in design.
      mask Display:
      | NxtrConf = 'Nexteer Confidential';
      | 
      | sys = bdroot; %handle for the current model ("system")
      | first = get_param(sys,'Created');
      | if(isempty(first))
      |     first = datestr(now,'yyyy');
      | else
      |     first = first(end-3:end);  %year is last four digits
      | end
      | 
      | last = get_param(sys,'LastModifiedDate');
      | if isempty(last)
      |     last = datestr(now,'yyyy');
      | else
      |     last = last(end-3:end);
      | end
      | 
      | if strcmp(first,last)
      |     fprintf('%s -- Copyright %s Nexteer',NxtrConf,first)
      | else
      |     fprintf('%s -- %s%s- %s Nexteer',NxtrConf,char(169),first,last)
      | end
  "EnhdQuadDampg " : Subsystem
  MotVelBasdDampg : Subsystem
  Product : Product  RequirementInfo={'linktype_rmi_doors' '0000a525 (/E-STEER Core/SubSystem Specifications/Application Functions/SF003A Damping)' '#SF003A_118' 'true' 'REQ: SF003A_118' '' } %GIDa_c8908fde_3bcd_4fbf_bd3a_e03923d152e8  Inputs=3  RndMeth=Zero
  MotVelDampg : Outport
  wires:
  HwTq/1 -> "EnhdQuadDampg "/1(HwTq)
  MotVelBasdDampg/1(MotVelDampgCmd) -> Product/3
  "EnhdQuadDampg "/1(QuadDampgSca) -> Product/1
  Product/1 -> MotVelDampg/1  "ActvDampg"
  TSca/1 -> Product/2
  MotVelCrf/1 -> [MotVelCrf]
  [MotVelCrf] -> "EnhdQuadDampg "/2(MotVelCrf)
  [MotVelCrf] -> MotVelBasdDampg/1(MotVelCrf)
  VehSpd/1 -> MotVelBasdDampg/2(VehSpd)

== system SF003A_Dampg/Dampg/DampgPer1/CmdDiChk/CopyRight2 ==

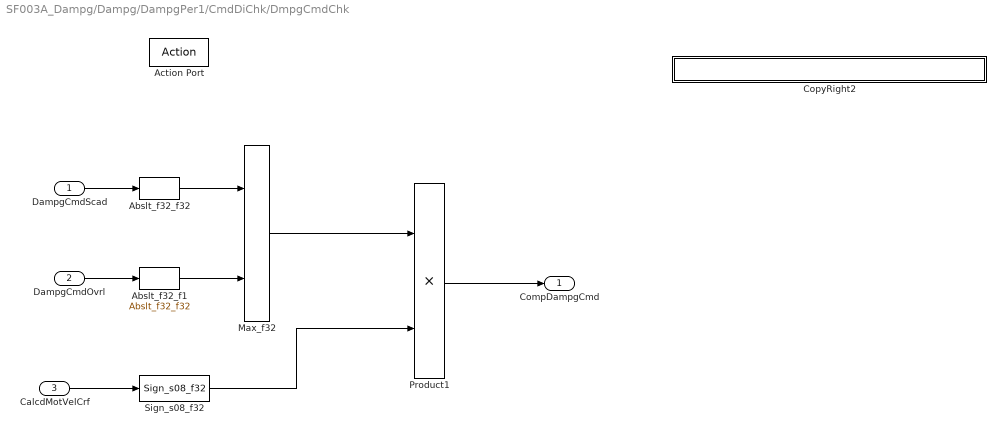
== system SF003A_Dampg/Dampg/DampgPer1/CmdDiChk/DmpgCmdChk ==
  DampgCmdScad : Inport
  DampgCmdOvrl : Inport  Port=2
  CalcdMotVelCrf : Inport  Port=3
  Action Port : ActionPort  ActionType=else
  Abslt_f32_f1 : NxtrAbslt/Abslt_f32_f32  RequirementInfo={'linktype_rmi_doors' '0000a525 (/E-STEER Core/SubSystem Specifications/Application Functions/SF003A Damping)' '#SF003A_128' 'true' 'REQ: SF003A_128' '' } %GIDa_b10d6be8_da84_4e3b_934f_c225b20cdb93  SFunctionSpec=single y1 = Abslt_f32_f32(single u1)
      settings: AttributesFormatString=%<Name>
  Abslt_f32_f32 : NxtrAbslt/Abslt_f32_f32  RequirementInfo={'linktype_rmi_doors' '0000a525 (/E-STEER Core/SubSystem Specifications/Application Functions/SF003A Damping)' '#SF003A_128' 'true' 'REQ: SF003A_128' '' } %GIDa_e74cdfb9_f095_4c11_8f8a_7f6d6693d9d6  SFunctionSpec=single y1 = Abslt_f32_f32(single u1)
      settings: AttributesFormatString=%<Name>
  CopyRight2 : Subsystem  Description=|  mask(Copyright Information){none=on}
      | Copyright info block.                                               
      |                                                                     
      | Place copyright information at the top of every subsystem in design.
      mask prompts: none "No parameters"
      mask help: Place copyright information at the top of every subsystem in design.
      mask Display:
      | NxtrConf = 'Nexteer Confidential';
      | 
      | sys = bdroot; %handle for the current model ("system")
      | first = get_param(sys,'Created');
      | if(isempty(first))
      |     first = datestr(now,'yyyy');
      | else
      |     first = first(end-3:end);  %year is last four digits
      | end
      | 
      | last = get_param(sys,'LastModifiedDate');
      | if isempty(last)
      |     last = datestr(now,'yyyy');
      | else
      |     last = last(end-3:end);
      | end
      | 
      | if strcmp(first,last)
      |     fprintf('%s -- Copyright %s Nexteer',NxtrConf,first)
      | else
      |     fprintf('%s -- %s%s- %s Nexteer',NxtrConf,char(169),first,last)
      | end
  Max_f32 : NxtrMax/Max_f32  RequirementInfo={'linktype_rmi_doors' '0000a525 (/E-STEER Core/SubSystem Specifications/Application Functions/SF003A Damping)' '#SF003A_128' 'true' 'REQ: SF003A_128' '' } %GIDa_cf4634e1_557d_43dc_88ca_431a3a2d2507  SFunctionSpec=single y1 = Max_f32(single u1, single u2)
      settings: AttributesFormatString=%<Name>
  Product1 : Product  RequirementInfo={'linktype_rmi_doors' '0000a525 (/E-STEER Core/SubSystem Specifications/Application Functions/SF003A Damping)' '#SF003A_129' 'true' 'REQ: SF003A_129' '' } %GIDa_cff8e35e_6814_42a0_ab97_6bbcbee1e48a  RndMeth=Zero
  Sign_s08_f32 : NxtrSign/Sign_s08_f32  RequirementInfo={'linktype_rmi_doors' '0000a525 (/E-STEER Core/SubSystem Specifications/Application Functions/SF003A Damping)' '#SF003A_129' 'true' 'REQ: SF003A_129' '' } %GIDa_e39c923e_f567_490b_9f6f_45e1fb18399e  SFunctionSpec=int8 y1 = Sign_s08_f32(single u1)
  CompDampgCmd : Outport
  wires:
  DampgCmdScad/1 -> Abslt_f32_f32/1
  Abslt_f32_f32/1 -> Max_f32/1
  Abslt_f32_f1/1 -> Max_f32/2
  Max_f32/1 -> Product1/1
  Sign_s08_f32/1 -> Product1/2
  DampgCmdOvrl/1 -> Abslt_f32_f1/1
  CalcdMotVelCrf/1 -> Sign_s08_f32/1
  Product1/1 -> CompDampgCmd/1

== system SF003A_Dampg/Dampg/DampgPer1/CmdDiChk/Zero_Command ==
  Action Port : ActionPort  ActionType=then
  Constant1 : Constant  RequirementInfo={} %GIDa_b06efe7e_48c8_49f6_a833_04aad4eae373  Value=0  OutDataTypeStr=single
  CopyRight2 : Subsystem  Description=|  mask(Copyright Information){none=on}
      | Copyright info block.                                               
      |                                                                     
      | Place copyright information at the top of every subsystem in design.
      mask prompts: none "No parameters"
      mask help: Place copyright information at the top of every subsystem in design.
      mask Display:
      | NxtrConf = 'Nexteer Confidential';
      | 
      | sys = bdroot; %handle for the current model ("system")
      | first = get_param(sys,'Created');
      | if(isempty(first))
      |     first = datestr(now,'yyyy');
      | else
      |     first = first(end-3:end);  %year is last four digits
      | end
      | 
      | last = get_param(sys,'LastModifiedDate');
      | if isempty(last)
      |     last = datestr(now,'yyyy');
      | else
      |     last = last(end-3:end);
      | end
      | 
      | if strcmp(first,last)
      |     fprintf('%s -- Copyright %s Nexteer',NxtrConf,first)
      | else
      |     fprintf('%s -- %s%s- %s Nexteer',NxtrConf,char(169),first,last)
      | end
  CompDampgCmd : Outport
  wires:
  Constant1/1 -> CompDampgCmd/1

== system SF003A_Dampg/Dampg/DampgPer1/FltInj - Sim/CopyRight2 ==

== system SF003A_Dampg/Dampg/DampgPer1/HydPwrSteerDampgCmd/CopyRight2 ==

== system SF003A_Dampg/Dampg/DampgPer1/MotVelDampgCmd/CopyRight2 ==
